simulink library "VIS_LIB"  (Simulink 8.6)
settings: Solver=ode45  StartTime=0.0  StopTime=10.0  RelTol=1e-3
undefined symbols (not defined in the file): AC, SIXOSEM_F_WD_AC_MASTER
libraries: cdsFilt x376, cdsEpicsOut x253, cdsEpicsIn x179, cdsTP x123, VIS_LIB x95, cdsMuxMatrix x91, cdsEpicsStringIn x75, cdsFiltCtrl x72, cdsFunctionCall x70, cdsRms x59, KAGRA_UTIL x25, STATE_BIO_MASTER x5
(part 16 of 38)

== system VIS_LIB/IpParts/TEST ==
  Ground1 : Ground
  Ground2 : Ground
  Ground3 : Ground
  L : cdsFilt/Subsystem  Tag=cdsFilt  Description=|
      | Purpose:                                                                                                                                                                                                                                  
      | Standard CDS IIR filter module.                                                                                                                                                                                                           
      |                                                                                                                                                                                                                                           
      | Operation:                                                                                                                                                                                                                                
      | Consists of 10 second order section IIR filters, plus a ramped gain stage. In FE code, also provides pre-defined test points and excitation channel inputs. The filter coefficients are defined in the LIGO system using the 'foton' tool.
      |                                                                                                                                                                                                                                           
      | Usage:                                                                                                                                                                                                                                    
      | Name the part with the desired filter module name.
      settings: AttributesFormatString=%<Tag>
  T : cdsFilt/Subsystem  Tag=cdsFilt  Description=|
      | Purpose:                                                                                                                                                                                                                                  
      | Standard CDS IIR filter module.                                                                                                                                                                                                           
      |                                                                                                                                                                                                                                           
      | Operation:                                                                                                                                                                                                                                
      | Consists of 10 second order section IIR filters, plus a ramped gain stage. In FE code, also provides pre-defined test points and excitation channel inputs. The filter coefficients are defined in the LIGO system using the 'foton' tool.
      |                                                                                                                                                                                                                                           
      | Usage:                                                                                                                                                                                                                                    
      | Name the part with the desired filter module name.
      settings: AttributesFormatString=%<Tag>
  Y : cdsFilt/Subsystem  Tag=cdsFilt  Description=|
      | Purpose:                                                                                                                                                                                                                                  
      | Standard CDS IIR filter module.                                                                                                                                                                                                           
      |                                                                                                                                                                                                                                           
      | Operation:                                                                                                                                                                                                                                
      | Consists of 10 second order section IIR filters, plus a ramped gain stage. In FE code, also provides pre-defined test points and excitation channel inputs. The filter coefficients are defined in the LIGO system using the 'foton' tool.
      |                                                                                                                                                                                                                                           
      | Usage:                                                                                                                                                                                                                                    
      | Name the part with the desired filter module name.
      settings: AttributesFormatString=%<Tag>
  LONG_Out : Outport
  TRANS_Out : Outport  Port=2
  YAW_Out : Outport  Port=3
  wires:
  Ground3/1 -> Y/1
  Ground2/1 -> T/1
  Ground1/1 -> L/1
  L/1 -> LONG_Out/1
  T/1 -> TRANS_Out/1
  Y/1 -> YAW_Out/1

== system VIS_LIB/IpParts/WD ==
  LVDT_H1_In : Inport
  LVDT_H2_In : Inport  Port=2
  LVDT_H3_In : Inport  Port=3
  ACC_H1_In : Inport  Port=4
  ACC_H2_In : Inport  Port=5
  ACC_H3_In : Inport  Port=6
  F0AC : Subsystem  AncestorBlock=SIXOSEM_F_WD_AC_MASTER/AC
  F0_AC_FLAG_Out : Outport
  wires:
  F0AC/1(FLAG) -> F0_AC_FLAG_Out/1
  LVDT_H1_In/1 -> F0AC/1(LVDT_H1_In)
  LVDT_H2_In/1 -> F0AC/2(LVDT_H2_In)
  LVDT_H3_In/1 -> F0AC/3(LVDT_H3_In)
  ACC_H1_In/1 -> F0AC/4(ACC_H1_In)
  ACC_H2_In/1 -> F0AC/5(ACC_H2_In1)
  ACC_H3_In/1 -> F0AC/6(ACC_H3_In1)

== system VIS_LIB/MODAL/GAS_MODE1 ==
  M1i : Inport
  M2i : Inport  Port=2
  M3i : Inport  Port=3
  M4i : Inport  Port=4
  M5i : Inport  Port=5
  TMP : Inport  Port=6
  TMY : Inport  Port=7
  ACT_FREQ : cdsEpicsIn/Subsystem  Tag=cdsEpicsIn  Description=|
      | Purpose:                                                                              
      | Create an EPICS input channel connection to the FE realtime controls.                 
      |                                                                                       
      | Operation:                                                                            
      | Outputs value from an EPICS ai record. Value is floating point with a precision of 3..
      |                                                                                       
      | Usage:                                                                                
      | Name the part with the desired EPICS channel name.
      settings: AttributesFormatString=%<Tag>
  ACT_PHASE_SHIFT : Subsystem
  Demux : Demux  Outputs=1
  Demux2 : Demux  Outputs=5
  GAS_ACT_VECTOR : cdsRampMuxMatrix/Subsystem  Tag=cdsRampMuxMatrix
      settings: AttributesFormatString=%<Tag>
  Mux : Mux  Inputs=7
  Mux1 : Mux  Inputs=1
  SENS_FREQ : cdsEpicsIn/Subsystem  Tag=cdsEpicsIn  Description=|
      | Purpose:                                                                              
      | Create an EPICS input channel connection to the FE realtime controls.                 
      |                                                                                       
      | Operation:                                                                            
      | Outputs value from an EPICS ai record. Value is floating point with a precision of 3..
      |                                                                                       
      | Usage:                                                                                
      | Name the part with the desired EPICS channel name.
      settings: AttributesFormatString=%<Tag>
  SENS_PHASE_SHIFT : Subsystem
  SENS_VECTOR : cdsMuxMatrix/Subsystem  Tag=cdsMuxMatrix  Description=Any size matrix. Inputs and outputs must be connected using Mux and Demux parts.
      settings: AttributesFormatString=%<Tag>
  SERVO : cdsFilt/Subsystem  Tag=cdsFilt  Description=|
      | Purpose:                                                                                                                                                                                                                                  
      | Standard CDS IIR filter module.                                                                                                                                                                                                           
      |                                                                                                                                                                                                                                           
      | Operation:                                                                                                                                                                                                                                
      | Consists of 10 second order section IIR filters, plus a ramped gain stage. In FE code, also provides pre-defined test points and excitation channel inputs. The filter coefficients are defined in the LIGO system using the 'foton' tool.
      |                                                                                                                                                                                                                                           
      | Usage:                                                                                                                                                                                                                                    
      | Name the part with the desired filter module name.
      settings: AttributesFormatString=%<Tag>
  M1 : Outport
  M2 : Outport  Port=2
  M3 : Outport  Port=3
  M4 : Outport  Port=4
  M5 : Outport  Port=5
  wires:
  TMP/1 -> SENS_PHASE_SHIFT/6(In6)
  M5i/1 -> SENS_PHASE_SHIFT/5(In5)
  TMY/1 -> SENS_PHASE_SHIFT/7(In7)
  M3i/1 -> SENS_PHASE_SHIFT/3(In3)
  M4i/1 -> SENS_PHASE_SHIFT/4(In4)
  M2i/1 -> SENS_PHASE_SHIFT/2(In2)
  M1i/1 -> SENS_PHASE_SHIFT/1(In1)
  SENS_PHASE_SHIFT/7(Out7) -> Mux/7
  SENS_PHASE_SHIFT/6(Out6) -> Mux/6
  SENS_PHASE_SHIFT/5(Out5) -> Mux/5
  SENS_PHASE_SHIFT/4(Out4) -> Mux/4
  SENS_PHASE_SHIFT/3(Out3) -> Mux/3
  SENS_PHASE_SHIFT/2(Out2) -> Mux/2
  SENS_PHASE_SHIFT/1(Out1) -> Mux/1
  SENS_FREQ/1 -> SENS_PHASE_SHIFT/8(Freq)
  Mux/1 -> SENS_VECTOR/1
  SENS_VECTOR/1 -> Demux/1
  Demux/1 -> SERVO/1
  Mux1/1 -> GAS_ACT_VECTOR/1
  SERVO/1 -> Mux1/1
  ACT_PHASE_SHIFT/1(Out1) -> M1/1
  ACT_PHASE_SHIFT/2(Out2) -> M2/1
  ACT_PHASE_SHIFT/3(Out3) -> M3/1
  ACT_PHASE_SHIFT/4(Out4) -> M4/1
  ACT_PHASE_SHIFT/5(Out5) -> M5/1
  GAS_ACT_VECTOR/1 -> Demux2/1
  Demux2/1 -> ACT_PHASE_SHIFT/1(In1)
  Demux2/2 -> ACT_PHASE_SHIFT/2(In2)
  Demux2/3 -> ACT_PHASE_SHIFT/3(In3)
  Demux2/4 -> ACT_PHASE_SHIFT/4(In4)
  Demux2/5 -> ACT_PHASE_SHIFT/5(In5)
  ACT_FREQ/1 -> ACT_PHASE_SHIFT/6(Freq)

== system VIS_LIB/MODAL/GAS_MODE_PARAMS ==
  CP_COEF : Subsystem
  DECAY_TIME : cdsEpicsIn/Subsystem  Tag=cdsEpicsIn  Description=|
      | Purpose:                                                                              
      | Create an EPICS input channel connection to the FE realtime controls.                 
      |                                                                                       
      | Operation:                                                                            
      | Outputs value from an EPICS ai record. Value is floating point with a precision of 3..
      |                                                                                       
      | Usage:                                                                                
      | Name the part with the desired EPICS channel name.
      settings: AttributesFormatString=%<Tag>
  DEGEN_MODE : cdsEpicsStringIn/EpicsStringIn  Tag=cdsEpicsStringIn  Description=cdsEpicsStringIn
      settings: AttributesFormatString=%<Tag>
  DOF : cdsEpicsStringIn/EpicsStringIn  Tag=cdsEpicsStringIn  Description=cdsEpicsStringIn
      settings: AttributesFormatString=%<Tag>
  FREQ : cdsEpicsIn/Subsystem  Tag=cdsEpicsIn  Description=|
      | Purpose:                                                                              
      | Create an EPICS input channel connection to the FE realtime controls.                 
      |                                                                                       
      | Operation:                                                                            
      | Outputs value from an EPICS ai record. Value is floating point with a precision of 3..
      |                                                                                       
      | Usage:                                                                                
      | Name the part with the desired EPICS channel name.
      settings: AttributesFormatString=%<Tag>
  Ground{,1..3} (4 alike) : Ground
  MEAS_DATE : Subsystem
  PLL_SENS : cdsEpicsStringIn/EpicsStringIn  Tag=cdsEpicsStringIn  Description=cdsEpicsStringIn
      settings: AttributesFormatString=%<Tag>
  PRE_FREQ : cdsEpicsIn/Subsystem  Tag=cdsEpicsIn  Description=|
      | Purpose:                                                                              
      | Create an EPICS input channel connection to the FE realtime controls.                 
      |                                                                                       
      | Operation:                                                                            
      | Outputs value from an EPICS ai record. Value is floating point with a precision of 3..
      |                                                                                       
      | Usage:                                                                                
      | Name the part with the desired EPICS channel name.
      settings: AttributesFormatString=%<Tag>
  PRE_Q : cdsEpicsIn/Subsystem  Tag=cdsEpicsIn  Description=|
      | Purpose:                                                                              
      | Create an EPICS input channel connection to the FE realtime controls.                 
      |                                                                                       
      | Operation:                                                                            
      | Outputs value from an EPICS ai record. Value is floating point with a precision of 3..
      |                                                                                       
      | Usage:                                                                                
      | Name the part with the desired EPICS channel name.
      settings: AttributesFormatString=%<Tag>
  Q_VAL : cdsEpicsIn/Subsystem  Tag=cdsEpicsIn  Description=|
      | Purpose:                                                                              
      | Create an EPICS input channel connection to the FE realtime controls.                 
      |                                                                                       
      | Operation:                                                                            
      | Outputs value from an EPICS ai record. Value is floating point with a precision of 3..
      |                                                                                       
      | Usage:                                                                                
      | Name the part with the desired EPICS channel name.
      settings: AttributesFormatString=%<Tag>
  REL_PHASE : Subsystem
  TM : Subsystem
  Terminator{1..4,12} (5 alike) : Terminator
  USER_DESCRIPTION : cdsEpicsStringIn/EpicsStringIn  Tag=cdsEpicsStringIn  Description=cdsEpicsStringIn
      settings: AttributesFormatString=%<Tag>
  wires:
  Ground3/1 -> DEGEN_MODE/1
  Ground/1 -> DOF/1
  Ground1/1 -> USER_DESCRIPTION/1
  FREQ/1 -> Terminator12/1
  Q_VAL/1 -> Terminator1/1
  DECAY_TIME/1 -> Terminator2/1
  PRE_FREQ/1 -> Terminator3/1
  PRE_Q/1 -> Terminator4/1
  Ground2/1 -> PLL_SENS/1

== system VIS_LIB/MODAL/MODE1 ==
  IPL : Inport
  IPT : Inport  Port=2
  IPV : Inport  Port=3
  IPR : Inport  Port=4
  IPP : Inport  Port=5
  IPY : Inport  Port=6
  BFL : Inport  Port=7
  BFT : Inport  Port=8
  BFV : Inport  Port=9
  BFR : Inport  Port=10
  BFP : Inport  Port=11
  BFY : Inport  Port=12
  MNL : Inport  Port=13
  MNT : Inport  Port=14
  MNV : Inport  Port=15
  MNR : Inport  Port=16
  MNP : Inport  Port=17
  MNY : Inport  Port=18
  IML : Inport  Port=19
  IMT : Inport  Port=20
  IMV : Inport  Port=21
  IMR : Inport  Port=22
  IMP : Inport  Port=23
  IMY : Inport  Port=24
  TML : Inport  Port=25
  TMT : Inport  Port=26
  TMV : Inport  Port=27
  TMR : Inport  Port=28
  TMP : Inport  Port=29
  TMY : Inport  Port=30
  ACT_FREQ : cdsEpicsIn/Subsystem  Tag=cdsEpicsIn  Description=|
      | Purpose:                                                                              
      | Create an EPICS input channel connection to the FE realtime controls.                 
      |                                                                                       
      | Operation:                                                                            
      | Outputs value from an EPICS ai record. Value is floating point with a precision of 3..
      |                                                                                       
      | Usage:                                                                                
      | Name the part with the desired EPICS channel name.
      settings: AttributesFormatString=%<Tag>
  ACT_PHASE_SHIFT : Subsystem
  BF_ACT_VECTOR : cdsMuxMatrix/Subsystem  Tag=cdsMuxMatrix  Description=Any size matrix. Inputs and outputs must be connected using Mux and Demux parts.
      settings: AttributesFormatString=%<Tag>
  Demux : Demux  Outputs=1
  Demux1 : Demux  Outputs=3
  Demux2 : Demux  Outputs=5
  Demux3 : Demux  Outputs=6
  Demux4 : Demux  Outputs=6
  Demux5 : Demux  Outputs=6
  Demux6 : Demux  Outputs=3
  IM_ACT_VECTOR : cdsMuxMatrix/Subsystem  Tag=cdsMuxMatrix  Description=Any size matrix. Inputs and outputs must be connected using Mux and Demux parts.
      settings: AttributesFormatString=%<Tag>
  IP_ACT_VECTOR : cdsMuxMatrix/Subsystem  Tag=cdsMuxMatrix  Description=Any size matrix. Inputs and outputs must be connected using Mux and Demux parts.
      settings: AttributesFormatString=%<Tag>
  MN_ACT_VECTOR : cdsMuxMatrix/Subsystem  Tag=cdsMuxMatrix  Description=Any size matrix. Inputs and outputs must be connected using Mux and Demux parts.
      settings: AttributesFormatString=%<Tag>
  Mux : Mux  Inputs=30
  Mux{1..6} (6 alike) : Mux  Inputs=1
  SENS_FREQ : cdsEpicsIn/Subsystem  Tag=cdsEpicsIn  Description=|
      | Purpose:                                                                              
      | Create an EPICS input channel connection to the FE realtime controls.                 
      |                                                                                       
      | Operation:                                                                            
      | Outputs value from an EPICS ai record. Value is floating point with a precision of 3..
      |                                                                                       
      | Usage:                                                                                
      | Name the part with the desired EPICS channel name.
      settings: AttributesFormatString=%<Tag>
  SENS_PHASE_SHIFT : Subsystem
  SENS_VECTOR : cdsMuxMatrix/Subsystem  Tag=cdsMuxMatrix  Description=Any size matrix. Inputs and outputs must be connected using Mux and Demux parts.
      settings: AttributesFormatString=%<Tag>
  SERVO : cdsFilt/Subsystem  Tag=cdsFilt  Description=|
      | Purpose:                                                                                                                                                                                                                                  
      | Standard CDS IIR filter module.                                                                                                                                                                                                           
      |                                                                                                                                                                                                                                           
      | Operation:                                                                                                                                                                                                                                
      | Consists of 10 second order section IIR filters, plus a ramped gain stage. In FE code, also provides pre-defined test points and excitation channel inputs. The filter coefficients are defined in the LIGO system using the 'foton' tool.
      |                                                                                                                                                                                                                                           
      | Usage:                                                                                                                                                                                                                                    
      | Name the part with the desired filter module name.
      settings: AttributesFormatString=%<Tag>
  STAGE_DIVIDER : cdsRampMuxMatrix/Subsystem  Tag=cdsRampMuxMatrix
      settings: AttributesFormatString=%<Tag>
  TM_ACT_VECTOR : cdsMuxMatrix/Subsystem  Tag=cdsMuxMatrix  Description=Any size matrix. Inputs and outputs must be connected using Mux and Demux parts.
      settings: AttributesFormatString=%<Tag>
  IPLo : Outport
  IPTo : Outport  Port=2
  IPYo : Outport  Port=3
  BFLo : Outport  Port=4
  BFTo : Outport  Port=5
  BFVo : Outport  Port=6
  BFRo : Outport  Port=7
  BFPo : Outport  Port=8
  BFYo : Outport  Port=9
  MNLo : Outport  Port=10
  MNTo : Outport  Port=11
  MNVo : Outport  Port=12
  MNRo : Outport  Port=13
  MNPo : Outport  Port=14
  MNYo : Outport  Port=15
  IMLo : Outport  Port=16
  IMTo : Outport  Port=17
  IMVo : Outport  Port=18
  IMRo : Outport  Port=19
  IMPo : Outport  Port=20
  IMYo : Outport  Port=21
  TMLo : Outport  Port=22
  TMPo : Outport  Port=23
  TMYo : Outport  Port=24
  wires:
  Demux2/5 -> Mux6/1
  Demux2/4 -> Mux5/1
  Demux2/3 -> Mux4/1
  Demux2/2 -> Mux3/1
  Demux2/1 -> Mux2/1
  Demux6/3 -> ACT_PHASE_SHIFT/24(In24)
  Demux6/2 -> ACT_PHASE_SHIFT/23(In23)
  Demux6/1 -> ACT_PHASE_SHIFT/22(In22)
  Mux6/1 -> TM_ACT_VECTOR/1
  TM_ACT_VECTOR/1 -> Demux6/1
  Demux5/6 -> ACT_PHASE_SHIFT/21(In21)
  Demux5/5 -> ACT_PHASE_SHIFT/20(In20)
  Demux5/4 -> ACT_PHASE_SHIFT/19(In19)
  Demux5/2 -> ACT_PHASE_SHIFT/17(In17)
  Demux5/3 -> ACT_PHASE_SHIFT/18(In18)
  Demux5/1 -> ACT_PHASE_SHIFT/16(In16)
  Mux5/1 -> IM_ACT_VECTOR/1
  IM_ACT_VECTOR/1 -> Demux5/1
  Demux4/6 -> ACT_PHASE_SHIFT/15(In15)
  Demux4/5 -> ACT_PHASE_SHIFT/14(In14)
  Demux4/4 -> ACT_PHASE_SHIFT/13(In13)
  Demux4/2 -> ACT_PHASE_SHIFT/11(In11)
  Demux4/3 -> ACT_PHASE_SHIFT/12(In12)
  Demux4/1 -> ACT_PHASE_SHIFT/10(In10)
  Mux4/1 -> MN_ACT_VECTOR/1
  MN_ACT_VECTOR/1 -> Demux4/1
  Demux3/6 -> ACT_PHASE_SHIFT/9(In9)
  Demux3/5 -> ACT_PHASE_SHIFT/8(In8)
  Demux3/4 -> ACT_PHASE_SHIFT/7(In7)
  Demux3/2 -> ACT_PHASE_SHIFT/5(In5)
  Demux3/3 -> ACT_PHASE_SHIFT/6(In6)
  Demux3/1 -> ACT_PHASE_SHIFT/4(In4)
  Mux3/1 -> BF_ACT_VECTOR/1
  BF_ACT_VECTOR/1 -> Demux3/1
  Demux1/3 -> ACT_PHASE_SHIFT/3(In3)
  Demux1/2 -> ACT_PHASE_SHIFT/2(In2)
  Demux1/1 -> ACT_PHASE_SHIFT/1(In1)
  Mux2/1 -> IP_ACT_VECTOR/1
  STAGE_DIVIDER/1 -> Demux2/1
  ACT_FREQ/1 -> ACT_PHASE_SHIFT/25(Freq)
  ACT_PHASE_SHIFT/23(Out23) -> TMPo/1
  ACT_PHASE_SHIFT/22(Out22) -> TMLo/1
  ACT_PHASE_SHIFT/21(Out21) -> IMYo/1
  ACT_PHASE_SHIFT/20(Out20) -> IMPo/1
  ACT_PHASE_SHIFT/19(Out19) -> IMRo/1
  ACT_PHASE_SHIFT/18(Out18) -> IMVo/1
  ACT_PHASE_SHIFT/17(Out17) -> IMTo/1
  ACT_PHASE_SHIFT/16(Out16) -> IMLo/1
  ACT_PHASE_SHIFT/15(Out15) -> MNYo/1
  ACT_PHASE_SHIFT/14(Out14) -> MNPo/1
  ACT_PHASE_SHIFT/13(Out13) -> MNRo/1
  ACT_PHASE_SHIFT/12(Out12) -> MNVo/1
  ACT_PHASE_SHIFT/11(Out11) -> MNTo/1
  ACT_PHASE_SHIFT/10(Out10) -> MNLo/1
  ACT_PHASE_SHIFT/9(Out9) -> BFYo/1
  ACT_PHASE_SHIFT/8(Out8) -> BFPo/1
  ACT_PHASE_SHIFT/7(Out7) -> BFRo/1
  ACT_PHASE_SHIFT/6(Out6) -> BFVo/1
  ACT_PHASE_SHIFT/5(Out5) -> BFTo/1
  ACT_PHASE_SHIFT/4(Out4) -> BFLo/1
  ACT_PHASE_SHIFT/3(Out3) -> IPYo/1
  ACT_PHASE_SHIFT/2(Out2) -> IPTo/1
  ACT_PHASE_SHIFT/1(Out1) -> IPLo/1
  ACT_PHASE_SHIFT/24(Out24) -> TMYo/1
  SERVO/1 -> Mux1/1
  IP_ACT_VECTOR/1 -> Demux1/1
  Mux1/1 -> STAGE_DIVIDER/1
  Demux/1 -> SERVO/1
  SENS_VECTOR/1 -> Demux/1
  Mux/1 -> SENS_VECTOR/1
  SENS_FREQ/1 -> SENS_PHASE_SHIFT/31(Freq)
  SENS_PHASE_SHIFT/1(Out1) -> Mux/1
  SENS_PHASE_SHIFT/2(Out2) -> Mux/2
  SENS_PHASE_SHIFT/3(Out3) -> Mux/3
  SENS_PHASE_SHIFT/4(Out4) -> Mux/4
  SENS_PHASE_SHIFT/5(Out5) -> Mux/5
  SENS_PHASE_SHIFT/6(Out6) -> Mux/6
  SENS_PHASE_SHIFT/7(Out7) -> Mux/7
  SENS_PHASE_SHIFT/8(Out8) -> Mux/8
  SENS_PHASE_SHIFT/9(Out9) -> Mux/9
  SENS_PHASE_SHIFT/10(Out10) -> Mux/10
  SENS_PHASE_SHIFT/11(Out11) -> Mux/11
  SENS_PHASE_SHIFT/12(Out12) -> Mux/12
  SENS_PHASE_SHIFT/13(Out13) -> Mux/13
  SENS_PHASE_SHIFT/14(Out14) -> Mux/14
  SENS_PHASE_SHIFT/15(Out15) -> Mux/15
  SENS_PHASE_SHIFT/16(Out16) -> Mux/16
  SENS_PHASE_SHIFT/17(Out17) -> Mux/17
  SENS_PHASE_SHIFT/18(Out18) -> Mux/18
  SENS_PHASE_SHIFT/19(Out19) -> Mux/19
  SENS_PHASE_SHIFT/20(Out20) -> Mux/20
  SENS_PHASE_SHIFT/21(Out21) -> Mux/21
  SENS_PHASE_SHIFT/22(Out22) -> Mux/22
  SENS_PHASE_SHIFT/23(Out23) -> Mux/23
  SENS_PHASE_SHIFT/24(Out24) -> Mux/24
  IPL/1 -> SENS_PHASE_SHIFT/1(In1)
  IPT/1 -> SENS_PHASE_SHIFT/2(In2)
  IPR/1 -> SENS_PHASE_SHIFT/4(In4)
  IPV/1 -> SENS_PHASE_SHIFT/3(In3)
  BFL/1 -> SENS_PHASE_SHIFT/7(In7)
  IPP/1 -> SENS_PHASE_SHIFT/5(In5)
  IPY/1 -> SENS_PHASE_SHIFT/6(In6)
  IMP/1 -> SENS_PHASE_SHIFT/23(In23)
  BFT/1 -> SENS_PHASE_SHIFT/8(In8)
  BFV/1 -> SENS_PHASE_SHIFT/9(In9)
  BFR/1 -> SENS_PHASE_SHIFT/10(In10)
  BFP/1 -> SENS_PHASE_SHIFT/11(In11)
  BFY/1 -> SENS_PHASE_SHIFT/12(In12)
  MNL/1 -> SENS_PHASE_SHIFT/13(In13)
  MNT/1 -> SENS_PHASE_SHIFT/14(In14)
  MNV/1 -> SENS_PHASE_SHIFT/15(In15)
  MNR/1 -> SENS_PHASE_SHIFT/16(In16)
  MNP/1 -> SENS_PHASE_SHIFT/17(In17)
  MNY/1 -> SENS_PHASE_SHIFT/18(In18)
  IML/1 -> SENS_PHASE_SHIFT/19(In19)
  IMT/1 -> SENS_PHASE_SHIFT/20(In20)
  IMV/1 -> SENS_PHASE_SHIFT/21(In21)
  IMR/1 -> SENS_PHASE_SHIFT/22(In22)
  IMY/1 -> SENS_PHASE_SHIFT/24(In24)
  TML/1 -> SENS_PHASE_SHIFT/25(In25)
  TMY/1 -> SENS_PHASE_SHIFT/30(In30)
  TMP/1 -> SENS_PHASE_SHIFT/29(In29)
  TMV/1 -> SENS_PHASE_SHIFT/27(In27)
  TMT/1 -> SENS_PHASE_SHIFT/26(In26)
  TMR/1 -> SENS_PHASE_SHIFT/28(In28)
  SENS_PHASE_SHIFT/25(Out25) -> Mux/25
  SENS_PHASE_SHIFT/26(Out26) -> Mux/26
  SENS_PHASE_SHIFT/27(Out27) -> Mux/27
  SENS_PHASE_SHIFT/28(Out28) -> Mux/28
  SENS_PHASE_SHIFT/29(Out29) -> Mux/29
  SENS_PHASE_SHIFT/30(Out30) -> Mux/30

== system VIS_LIB/MODAL/MODE_PARAMS ==
  BF : Subsystem
  CP_COEF : Subsystem
  DECAY_TIME : cdsEpicsIn/Subsystem  Tag=cdsEpicsIn  Description=|
      | Purpose:                                                                              
      | Create an EPICS input channel connection to the FE realtime controls.                 
      |                                                                                       
      | Operation:                                                                            
      | Outputs value from an EPICS ai record. Value is floating point with a precision of 3..
      |                                                                                       
      | Usage:                                                                                
      | Name the part with the desired EPICS channel name.
      settings: AttributesFormatString=%<Tag>
  DEGEN_MODE : cdsEpicsStringIn/EpicsStringIn  Tag=cdsEpicsStringIn  Description=cdsEpicsStringIn
      settings: AttributesFormatString=%<Tag>
  DOF : cdsEpicsStringIn/EpicsStringIn  Tag=cdsEpicsStringIn  Description=cdsEpicsStringIn
      settings: AttributesFormatString=%<Tag>
  FREQ : cdsEpicsIn/Subsystem  Tag=cdsEpicsIn  Description=|
      | Purpose:                                                                              
      | Create an EPICS input channel connection to the FE realtime controls.                 
      |                                                                                       
      | Operation:                                                                            
      | Outputs value from an EPICS ai record. Value is floating point with a precision of 3..
      |                                                                                       
      | Usage:                                                                                
      | Name the part with the desired EPICS channel name.
      settings: AttributesFormatString=%<Tag>
  Ground{,1..3} (4 alike) : Ground
  IM : Subsystem
  IP : Subsystem
  MEAS_DATE : Subsystem
  MN : Subsystem
  PLL_SENS : cdsEpicsStringIn/EpicsStringIn  Tag=cdsEpicsStringIn  Description=cdsEpicsStringIn
      settings: AttributesFormatString=%<Tag>
  PRE_FREQ : cdsEpicsIn/Subsystem  Tag=cdsEpicsIn  Description=|
      | Purpose:                                                                              
      | Create an EPICS input channel connection to the FE realtime controls.                 
      |                                                                                       
      | Operation:                                                                            
      | Outputs value from an EPICS ai record. Value is floating point with a precision of 3..
      |                                                                                       
      | Usage:                                                                                
      | Name the part with the desired EPICS channel name.
      settings: AttributesFormatString=%<Tag>
  PRE_Q : cdsEpicsIn/Subsystem  Tag=cdsEpicsIn  Description=|
      | Purpose:                                                                              
      | Create an EPICS input channel connection to the FE realtime controls.                 
      |                                                                                       
      | Operation:                                                                            
      | Outputs value from an EPICS ai record. Value is floating point with a precision of 3..
      |                                                                                       
      | Usage:                                                                                
      | Name the part with the desired EPICS channel name.
      settings: AttributesFormatString=%<Tag>
  Q_VAL : cdsEpicsIn/Subsystem  Tag=cdsEpicsIn  Description=|
      | Purpose:                                                                              
      | Create an EPICS input channel connection to the FE realtime controls.                 
      |                                                                                       
      | Operation:                                                                            
      | Outputs value from an EPICS ai record. Value is floating point with a precision of 3..
      |                                                                                       
      | Usage:                                                                                
      | Name the part with the desired EPICS channel name.
      settings: AttributesFormatString=%<Tag>
  REL_PHASE : Subsystem
  TM : Subsystem
  Terminator{1..4,12} (5 alike) : Terminator
  USER_DESCRIPTION : cdsEpicsStringIn/EpicsStringIn  Tag=cdsEpicsStringIn  Description=cdsEpicsStringIn
      settings: AttributesFormatString=%<Tag>
  wires:
  Ground3/1 -> DEGEN_MODE/1
  Ground/1 -> DOF/1
  Ground1/1 -> USER_DESCRIPTION/1
  FREQ/1 -> Terminator12/1
  Q_VAL/1 -> Terminator1/1
  DECAY_TIME/1 -> Terminator2/1
  PRE_FREQ/1 -> Terminator3/1
  PRE_Q/1 -> Terminator4/1
  Ground2/1 -> PLL_SENS/1

== system VIS_LIB/MODAL/MODE_PARAMS1 ==
  DECAY_TIME : cdsEpicsIn/Subsystem  Tag=cdsEpicsIn  Description=|
      | Purpose:                                                                              
      | Create an EPICS input channel connection to the FE realtime controls.                 
      |                                                                                       
      | Operation:                                                                            
      | Outputs value from an EPICS ai record. Value is floating point with a precision of 3..
      |                                                                                       
      | Usage:                                                                                
      | Name the part with the desired EPICS channel name.
      settings: AttributesFormatString=%<Tag>
  DEGEN_MODE : cdsEpicsStringIn/EpicsStringIn  Tag=cdsEpicsStringIn  Description=cdsEpicsStringIn
      settings: AttributesFormatString=%<Tag>
  DOF : cdsEpicsStringIn/EpicsStringIn  Tag=cdsEpicsStringIn  Description=cdsEpicsStringIn
      settings: AttributesFormatString=%<Tag>
  FREQ : cdsEpicsIn/Subsystem  Tag=cdsEpicsIn  Description=|
      | Purpose:                                                                              
      | Create an EPICS input channel connection to the FE realtime controls.                 
      |                                                                                       
      | Operation:                                                                            
      | Outputs value from an EPICS ai record. Value is floating point with a precision of 3..
      |                                                                                       
      | Usage:                                                                                
      | Name the part with the desired EPICS channel name.
      settings: AttributesFormatString=%<Tag>
  Ground{,1..3} (4 alike) : Ground
  MEAS_DATE : Subsystem
  PRE_FREQ : cdsEpicsIn/Subsystem  Tag=cdsEpicsIn  Description=|
      | Purpose:                                                                              
      | Create an EPICS input channel connection to the FE realtime controls.                 
      |                                                                                       
      | Operation:                                                                            
      | Outputs value from an EPICS ai record. Value is floating point with a precision of 3..
      |                                                                                       
      | Usage:                                                                                
      | Name the part with the desired EPICS channel name.
      settings: AttributesFormatString=%<Tag>
  PRE_Q : cdsEpicsIn/Subsystem  Tag=cdsEpicsIn  Description=|
      | Purpose:                                                                              
      | Create an EPICS input channel connection to the FE realtime controls.                 
      |                                                                                       
      | Operation:                                                                            
      | Outputs value from an EPICS ai record. Value is floating point with a precision of 3..
      |                                                                                       
      | Usage:                                                                                
      | Name the part with the desired EPICS channel name.
      settings: AttributesFormatString=%<Tag>
  Q_VAL : cdsEpicsIn/Subsystem  Tag=cdsEpicsIn  Description=|
      | Purpose:                                                                              
      | Create an EPICS input channel connection to the FE realtime controls.                 
      |                                                                                       
      | Operation:                                                                            
      | Outputs value from an EPICS ai record. Value is floating point with a precision of 3..
      |                                                                                       
      | Usage:                                                                                
      | Name the part with the desired EPICS channel name.
      settings: AttributesFormatString=%<Tag>
  SENSMAT : Subsystem
  STAGE : cdsEpicsStringIn/EpicsStringIn  Tag=cdsEpicsStringIn  Description=cdsEpicsStringIn
      settings: AttributesFormatString=%<Tag>
  STAGE_MOTION : Subsystem
  Terminator{1..4,12} (5 alike) : Terminator
  USER_DESCRIPTION : cdsEpicsStringIn/EpicsStringIn  Tag=cdsEpicsStringIn  Description=cdsEpicsStringIn
      settings: AttributesFormatString=%<Tag>
  wires:
  Ground3/1 -> DEGEN_MODE/1
  Ground/1 -> DOF/1
  Ground1/1 -> USER_DESCRIPTION/1
  FREQ/1 -> Terminator12/1
  Q_VAL/1 -> Terminator1/1
  DECAY_TIME/1 -> Terminator2/1
  PRE_FREQ/1 -> Terminator3/1
  PRE_Q/1 -> Terminator4/1
  Ground2/1 -> STAGE/1

== system VIS_LIB/MODAL/MODE_PARAMS1_GAS ==
  DECAY_TIME : cdsEpicsIn/Subsystem  Tag=cdsEpicsIn  Description=|
      | Purpose:                                                                              
      | Create an EPICS input channel connection to the FE realtime controls.                 
      |                                                                                       
      | Operation:                                                                            
      | Outputs value from an EPICS ai record. Value is floating point with a precision of 3..
      |                                                                                       
      | Usage:                                                                                
      | Name the part with the desired EPICS channel name.
      settings: AttributesFormatString=%<Tag>
  DEGEN_MODE : cdsEpicsStringIn/EpicsStringIn  Tag=cdsEpicsStringIn  Description=cdsEpicsStringIn
      settings: AttributesFormatString=%<Tag>
  DOF : cdsEpicsStringIn/EpicsStringIn  Tag=cdsEpicsStringIn  Description=cdsEpicsStringIn
      settings: AttributesFormatString=%<Tag>
  FREQ : cdsEpicsIn/Subsystem  Tag=cdsEpicsIn  Description=|
      | Purpose:                                                                              
      | Create an EPICS input channel connection to the FE realtime controls.                 
      |                                                                                       
      | Operation:                                                                            
      | Outputs value from an EPICS ai record. Value is floating point with a precision of 3..
      |                                                                                       
      | Usage:                                                                                
      | Name the part with the desired EPICS channel name.
      settings: AttributesFormatString=%<Tag>
  Ground{,1..3} (4 alike) : Ground
  MEAS_DATE : Subsystem
  PRE_FREQ : cdsEpicsIn/Subsystem  Tag=cdsEpicsIn  Description=|
      | Purpose:                                                                              
      | Create an EPICS input channel connection to the FE realtime controls.                 
      |                                                                                       
      | Operation:                                                                            
      | Outputs value from an EPICS ai record. Value is floating point with a precision of 3..
      |                                                                                       
      | Usage:                                                                                
      | Name the part with the desired EPICS channel name.
      settings: AttributesFormatString=%<Tag>
  PRE_Q : cdsEpicsIn/Subsystem  Tag=cdsEpicsIn  Description=|
      | Purpose:                                                                              
      | Create an EPICS input channel connection to the FE realtime controls.                 
      |                                                                                       
      | Operation:                                                                            
      | Outputs value from an EPICS ai record. Value is floating point with a precision of 3..
      |                                                                                       
      | Usage:                                                                                
      | Name the part with the desired EPICS channel name.
      settings: AttributesFormatString=%<Tag>
  Q_VAL : cdsEpicsIn/Subsystem  Tag=cdsEpicsIn  Description=|
      | Purpose:                                                                              
      | Create an EPICS input channel connection to the FE realtime controls.                 
      |                                                                                       
      | Operation:                                                                            
      | Outputs value from an EPICS ai record. Value is floating point with a precision of 3..
      |                                                                                       
      | Usage:                                                                                
      | Name the part with the desired EPICS channel name.
      settings: AttributesFormatString=%<Tag>
  SENSMAT : Subsystem
  STAGE : cdsEpicsStringIn/EpicsStringIn  Tag=cdsEpicsStringIn  Description=cdsEpicsStringIn
      settings: AttributesFormatString=%<Tag>
  STAGE_MOTION : Subsystem
  Terminator{1..4,12} (5 alike) : Terminator
  USER_DESCRIPTION : cdsEpicsStringIn/EpicsStringIn  Tag=cdsEpicsStringIn  Description=cdsEpicsStringIn
      settings: AttributesFormatString=%<Tag>
  wires:
  Ground3/1 -> DEGEN_MODE/1
  Ground/1 -> DOF/1
  Ground1/1 -> USER_DESCRIPTION/1
  FREQ/1 -> Terminator12/1
  Q_VAL/1 -> Terminator1/1
  DECAY_TIME/1 -> Terminator2/1
  PRE_FREQ/1 -> Terminator3/1
  PRE_Q/1 -> Terminator4/1
  Ground2/1 -> STAGE/1
